simulink model "ExampleThreePWMs"  (R2022b)
settings: Solver=VariableStepAuto  StartTime=0.0  StopTime=10.0  RelTol=1e-3
libraries: simulink x3, eePwmGeneratorThreeLevel x3, spsTriangleGeneratorLib x1
settings Model: Creator=uiv66426  LastModifiedBy=uiv66426

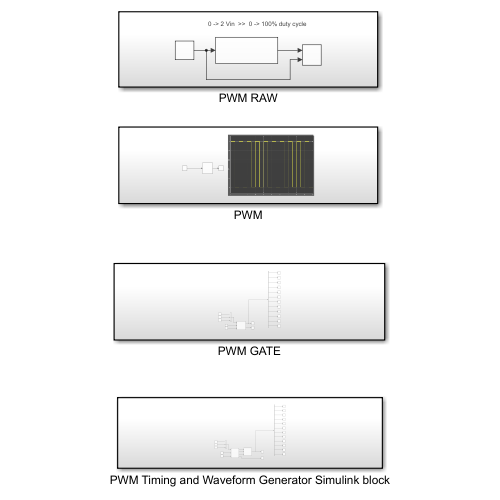
[thumbnail: Simulink's stored preview of the top-level diagram]
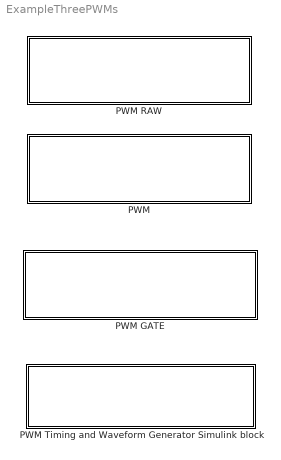
== system ExampleThreePWMs ==
  PWM : Subsystem
  PWM GATE : Subsystem
  PWM RAW : Subsystem
  PWM Timing and Waveform Generator Simulink block : Subsystem

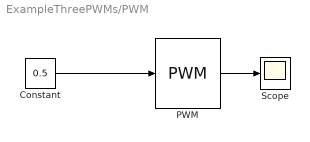
== system ExampleThreePWMs/PWM ==
  Constant : Constant  Value=0.5
  PWM : simulink/Discontinuities/PWM  DisableCoverage=on  Period=1  InitialDelay=0  DisallowZeroDutyCycle=off  RunAtFixedTimeIntervals=off  SampleTime=0.1
  Scope : Scope
  wires:
  Constant/1 -> PWM/1
  PWM/1 -> Scope/1

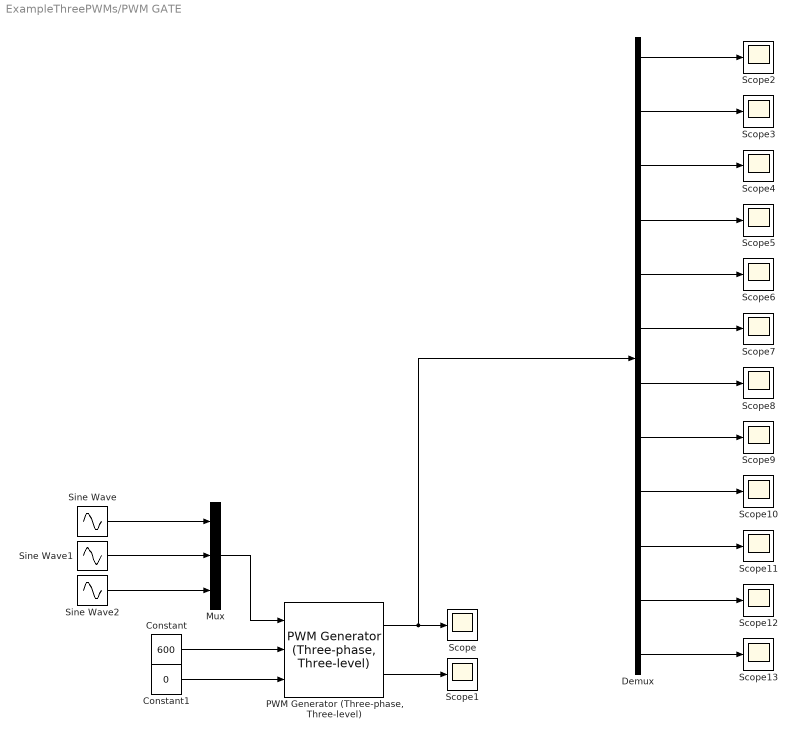
== system ExampleThreePWMs/PWM GATE ==
  Constant : Constant  Value=600
  Constant1 : Constant  Value=0
  Demux : Demux  Outputs=12
  Mux : Mux  Inputs=3
  "PWM Generator (Three-phase, Three-level)" : eePwmGeneratorThreeLevel/PWM Generator (Three-phase, Three-level)  CPWMMode=SPWM: sinusoidal PWM  fsw=1e3  Ts=5e-5
      settings: SamplingMode=Natural
      settings: LibrarySourceBlock=|
      | ee_sl_lib/Pulse Width
      | Modulation/PWM Generator
      | (Three-phase, Three-level)
  Scope{,1..13} (14 alike) : Scope
  Sine Wave : Sin  Frequency=50  SampleTime=0
  Sine Wave1 : Sin  Frequency=50  Phase=-120  SampleTime=0
  Sine Wave2 : Sin  Frequency=50  Phase=120  SampleTime=0
  wires:
  Constant1/1 -> "PWM Generator (Three-phase, Three-level)"/3
  "PWM Generator (Three-phase, Three-level)"/2 -> Scope1/1
  "PWM Generator (Three-phase, Three-level)"/1 -> Demux/1, Scope/1
  Sine Wave2/1 -> Mux/3
  Sine Wave1/1 -> Mux/2
  Mux/1 -> "PWM Generator (Three-phase, Three-level)"/1
  Constant/1 -> "PWM Generator (Three-phase, Three-level)"/2
  Sine Wave/1 -> Mux/1
  Demux/1 -> Scope2/1
  Demux/2 -> Scope3/1
  Demux/3 -> Scope4/1
  Demux/4 -> Scope5/1
  Demux/5 -> Scope6/1
  Demux/6 -> Scope7/1
  Demux/7 -> Scope8/1
  Demux/8 -> Scope9/1
  Demux/9 -> Scope10/1
  Demux/10 -> Scope11/1
  Demux/11 -> Scope12/1
  Demux/12 -> Scope13/1

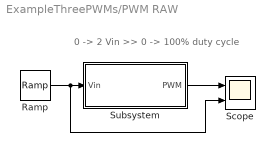
== system ExampleThreePWMs/PWM RAW ==
  note: 0 -> 2 Vin >> 0 -> 100% duty cycle
  Ramp : simulink/Sources/Ramp  slope=50  start=0  InitialOutput=-3
  Scope : Scope  NumInputPorts=2
  Subsystem : Subsystem
  wires:
  Subsystem/1(PWM) -> Scope/1
  Ramp/1 -> Subsystem/1(Vin), Scope/2

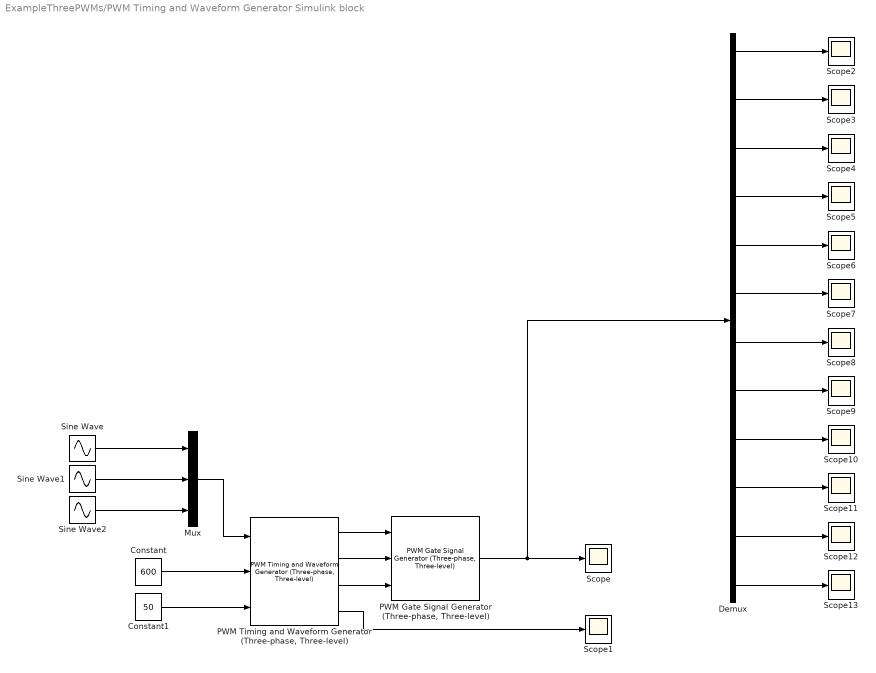
== system ExampleThreePWMs/PWM Timing and Waveform Generator Simulink block ==
  Constant : Constant  Value=600
  Constant1 : Constant  Value=50
  Demux : Demux  Outputs=12
  Mux : Mux  Inputs=3
  "PWM Gate Signal Generator (Three-phase, Three-level)" : eePwmGeneratorThreeLevel/PWM Gate Signal Generator (Three-phase, Three-level)  fsw=1e3  Ts=5e-5
      settings: SamplingMode=Natural
      settings: LibrarySourceBlock=|
      | ee_sl_lib/Pulse Width
      | Modulation/PWM Gate Signal Generator
      | (Three-phase, Three-level)
  "PWM Timing and Waveform Generator (Three-phase, Three-level)" : eePwmGeneratorThreeLevel/PWM Timing and Waveform Generator (Three-phase, Three-level)  CPWMMode=SPWM: sinusoidal PWM  fsw=1e3
      settings: SamplingMode=Natural
      settings: LibrarySourceBlock=|
      | ee_sl_lib/Pulse Width
      | Modulation/PWM Timing and Waveform
      | Generator
      | (Three-phase, Three-level)
  Scope{,1..13} (14 alike) : Scope
  Sine Wave : Sin  Frequency=50  SampleTime=0
  Sine Wave1 : Sin  Frequency=50  Phase=-120  SampleTime=0
  Sine Wave2 : Sin  Frequency=50  Phase=120  SampleTime=0
  wires:
  Sine Wave2/1 -> Mux/3
  Constant1/1 -> "PWM Timing and Waveform Generator (Three-phase, Three-level)"/3
  Mux/1 -> "PWM Timing and Waveform Generator (Three-phase, Three-level)"/1
  "PWM Timing and Waveform Generator (Three-phase, Three-level)"/1 -> "PWM Gate Signal Generator (Three-phase, Three-level)"/1
  Sine Wave1/1 -> Mux/2
  Constant/1 -> "PWM Timing and Waveform Generator (Three-phase, Three-level)"/2
  "PWM Gate Signal Generator (Three-phase, Three-level)"/1 -> Demux/1, Scope/1
  Sine Wave/1 -> Mux/1
  "PWM Timing and Waveform Generator (Three-phase, Three-level)"/2 -> "PWM Gate Signal Generator (Three-phase, Three-level)"/2
  "PWM Timing and Waveform Generator (Three-phase, Three-level)"/3 -> "PWM Gate Signal Generator (Three-phase, Three-level)"/3
  "PWM Timing and Waveform Generator (Three-phase, Three-level)"/4 -> Scope1/1
  Demux/2 -> Scope3/1
  Demux/7 -> Scope8/1
  Demux/12 -> Scope13/1
  Demux/1 -> Scope2/1
  Demux/10 -> Scope11/1
  Demux/3 -> Scope4/1
  Demux/5 -> Scope6/1
  Demux/6 -> Scope7/1
  Demux/8 -> Scope9/1
  Demux/4 -> Scope5/1
  Demux/9 -> Scope10/1
  Demux/11 -> Scope12/1

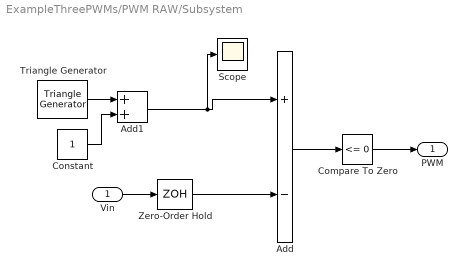
== system ExampleThreePWMs/PWM RAW/Subsystem ==
  Vin : Inport
  Add : Sum  Inputs=+-
  Add1 : Sum
  Compare To Zero : simulink/Logic and Bit Operations/Compare To Zero  relop=<=  OutDataTypeStr=boolean
  Constant : Constant
  Scope : Scope
  Triangle Generator : spsTriangleGeneratorLib/Triangle Generator  Freq=1e3  Phase=90  Ts=0
  Zero-Order Hold : ZeroOrderHold  SampleTime=-1
  PWM : Outport
  wires:
  Constant/1 -> Add1/2
  Add1/1 -> Add/1, Scope/1
  Triangle Generator/1 -> Add1/1
  Compare To Zero/1 -> PWM/1
  Add/1 -> Compare To Zero/1
  Zero-Order Hold/1 -> Add/2
  Vin/1 -> Zero-Order Hold/1
